simulink model "preg1_simu"  (R2021b)
settings: Solver=VariableStepAuto  StartTime=0.0  StopTime=15  RelTol=1e-3
values from neighbouring files (symbols this model uses):
  C = [21.53 -20.25]    [preg1.m]
  Gk = [0.6839 -0.7547;-0.2535 0.2798]    [preg1.m]
  Hk = [-0.01109;-0.01179]    [preg1.m]
  Hw = Hk    [preg1.m]
  K1 = K_21(end)    [preg1.m]
  K2 = K_21(1:end-1)    [preg1.m]
  Ke = acker(Gk',C',polos)'    [preg1.m]
  Ts = 0.4    [preg1.m]
settings Model: Creator=pierr  LastModifiedBy=catolica

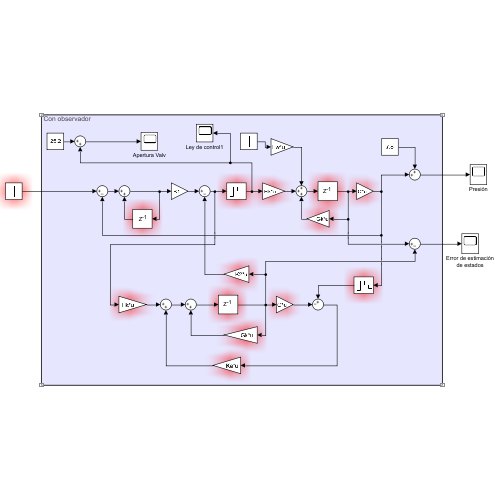
[thumbnail: Simulink's stored preview of the top-level diagram]
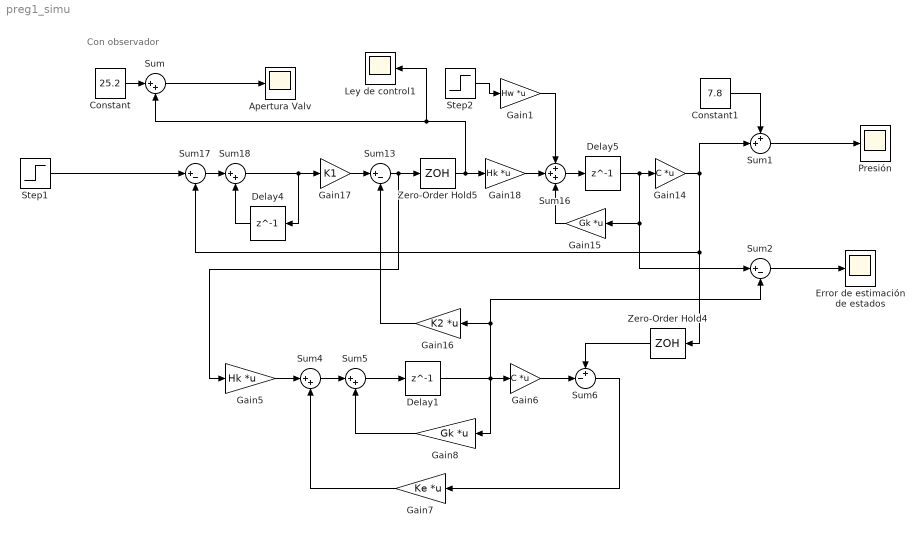
== system preg1_simu ==
  note: Con observador
  Apertura Valv : Scope
  Constant : Constant  Value=25.2
  Constant1 : Constant  Value=7.8
  Delay1 : Delay  DelayLength=1  SampleTime=Ts
  Delay4 : Delay  DelayLength=1  SampleTime=Ts
  Delay5 : Delay  DelayLength=1  InitialCondition=[0.1;0.1]  SampleTime=Ts
  Error de estimación de estados : Scope
  Gain1 : Gain  Gain=Hw  Multiplication=Matrix(K*u)
  Gain14 : Gain  Gain=C  Multiplication=Matrix(K*u)
  Gain15 : Gain  Gain=Gk  Multiplication=Matrix(K*u)
  Gain16 : Gain  Gain=K2  Multiplication=Matrix(K*u)
  Gain17 : Gain  Gain=K1
  Gain18 : Gain  Gain=Hk  Multiplication=Matrix(K*u)
  Gain5 : Gain  Gain=Hk  Multiplication=Matrix(K*u)
  Gain6 : Gain  Gain=C  Multiplication=Matrix(K*u)
  Gain7 : Gain  Gain=Ke  Multiplication=Matrix(K*u)
  Gain8 : Gain  Gain=Gk  Multiplication=Matrix(K*u)
  Ley de control1 : Scope
  Presión : Scope
  Step1 : Step  Time=0  After=10  SampleTime=Ts
  Step2 : Step  Time=0  After=-5  SampleTime=Ts
  Sum{,4..5,18} (4 alike) : Sum  Inputs=|++
  Sum1 : Sum  Inputs=++|
  Sum13 : Sum  Inputs=|+-
  Sum16 : Sum  Inputs=+++
  Sum17 : Sum  Inputs=|+-
  Sum2 : Sum  Inputs=|+-
  Sum6 : Sum  Inputs=+-|
  Zero-Order Hold4 : ZeroOrderHold  SampleTime=Ts
  Zero-Order Hold5 : ZeroOrderHold  SampleTime=Ts
  wires:
  Gain5/1 -> Sum4/1
  Sum4/1 -> Sum5/1
  Sum5/1 -> Delay1/1
  Delay1/1 -> Sum2/2, Gain16/1, Gain8/1, Gain6/1
  Gain6/1 -> Sum6/2
  Sum6/1 -> Gain7/1
  Gain8/1 -> Sum5/2
  Gain7/1 -> Sum4/2
  Sum16/1 -> Delay5/1
  Sum13/1 -> Gain5/1, Zero-Order Hold5/1
  Delay4/1 -> Sum18/2
  Gain16/1 -> Sum13/2
  Zero-Order Hold5/1 -> Sum/2, Ley de control1/1, Gain18/1
  Sum18/1 -> Delay4/1, Gain17/1
  Gain17/1 -> Sum13/1
  Sum17/1 -> Sum18/1
  Delay5/1 -> Gain14/1, Sum2/1, Gain15/1
  Zero-Order Hold4/1 -> Sum6/1
  Step2/1 -> Gain1/1
  Gain1/1 -> Sum16/1
  Gain15/1 -> Sum16/3
  Gain18/1 -> Sum16/2
  Constant/1 -> Sum/1
  Gain14/1 -> Sum17/2, Zero-Order Hold4/1, Sum1/2
  Sum1/1 -> Presión/1
  Constant1/1 -> Sum1/1
  Step1/1 -> Sum17/1
  Sum/1 -> Apertura Valv/1
  Sum2/1 -> Error de estimación de estados/1
